simulink model "cruise_control"  (R2021b)
settings: Solver=FixedStepAuto  StartTime=0.0  StopTime=50  RelTol=1e-3
undefined symbols (not defined in the file): b, m
settings Model: Creator=adish  LastModifiedBy=adish

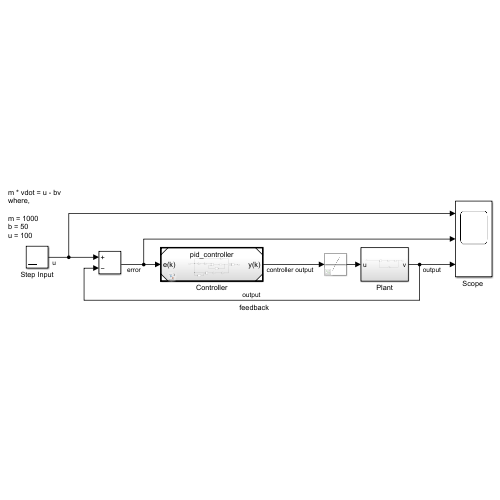
[thumbnail: Simulink's stored preview of the top-level diagram]
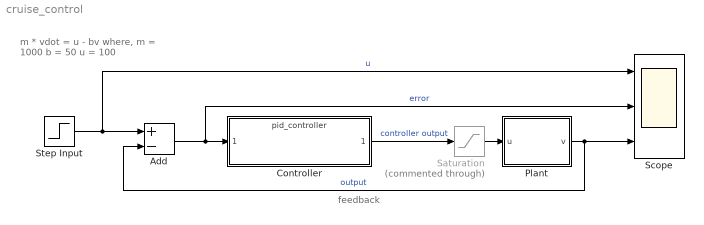
== system cruise_control ==
  note: feedback
  note: m * vdot = u - bv
      | where,
      |
      | m = 1000
      | b = 50
      | u = 100
  Add : Sum  Inputs=+-
  Controller : ModelReference  ModelNameDialog=pid_controller.slx  SimulationMode=Normal  ModelReferenceVersion=1.68
  Plant : Subsystem
  Saturation : Saturate  Commented=through  UpperLimit=300  LowerLimit=0
  "Scope " : Scope  NumInputPorts=3
  Step Input : Step  Time=2  After=u  SampleTime=0.01
  wires:
  Step Input/1 -> "Scope "/1, Add/1  "u"
  Plant/1(v) -> "Scope "/3, Add/2  "output"
  Add/1 -> Controller/1, "Scope "/2  "error"
  Controller/1 -> Saturation/1  "controller output"
  Saturation/1 -> Plant/1(u)

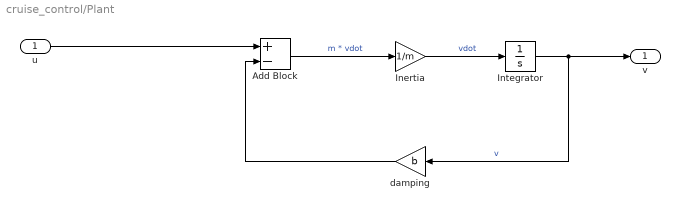
== system cruise_control/Plant ==
  u : Inport
  Add Block : Sum  Inputs=+-
  Inertia : Gain  Gain=1/m
  "Integrator " : Integrator
  damping : Gain  Gain=b
  v : Outport
  wires:
  Add Block/1 -> Inertia/1  "m * vdot"
  damping/1 -> Add Block/2
  Inertia/1 -> "Integrator "/1  "vdot"
  "Integrator "/1 -> v/1, damping/1  "v"
  u/1 -> Add Block/1
